simulink model "imu"  (R2014b)
settings: Solver=FixedStepDiscrete  StartTime=0.0  StopTime=inf  FixedStep=sample_time  RelTol=1e-3
settings Model: xpc_rtwmakecfg_data=_xpcethercatlib_  SimulationMode=external  BufferReuse=off  Creator=wmartin  LastModifiedBy=drl
settings SolverCC: EnableConcurrentExecution=on
settings DataIOCC: MaxDataPoints=1000000000  SaveFormat=StructureWithTime  SaveOutput=off  SaveTime=off
settings OptimizationCC: BlockReduction=off  OptimizeBlockIOStorage=off  BufferReuse=off  GlobalBufferReuse=off  ExpressionFolding=off  ExpressionDepthLimit=2147483647  LocalBlockOutputs=off  SimCompilerOptimization=On
settings DebuggingCC: ArtificialAlgebraicLoopMsg=none  UnderspecifiedInitializationDetection=Classic  MergeDetectMultiDrivingBlocksExec=none  StateNameClashWarn=warning
settings HardwareCC: ProdIntDivRoundTo=Zero  ProdEndianess=LittleEndian  ProdLongLongMode=on  ProdHWDeviceType=Generic->32-bit x86 compatible
settings ModelReferenceCC: EnableParallelModelReferenceBuilds=on  ModelReferenceNumInstancesAllowed=Single  ModelReferenceMinAlgLoopOccurrences=on
settings RTWCC: SystemTargetFile=slrt.tlc  TemplateMakefile=slrt_default_tmf  Description=Simulink Real-Time  RTWVerbose=off  ProcessScript=slrt_make_rtw_hook  RTWCompilerOptimization=On
settings CodeAppCC: MaxIdLength=256
settings SimulinkRealTimeCC: GeneratePreprocessorConditionals=Disable all  EnableShiftOperators=on  RL32LogBufSizeModifier=100000000

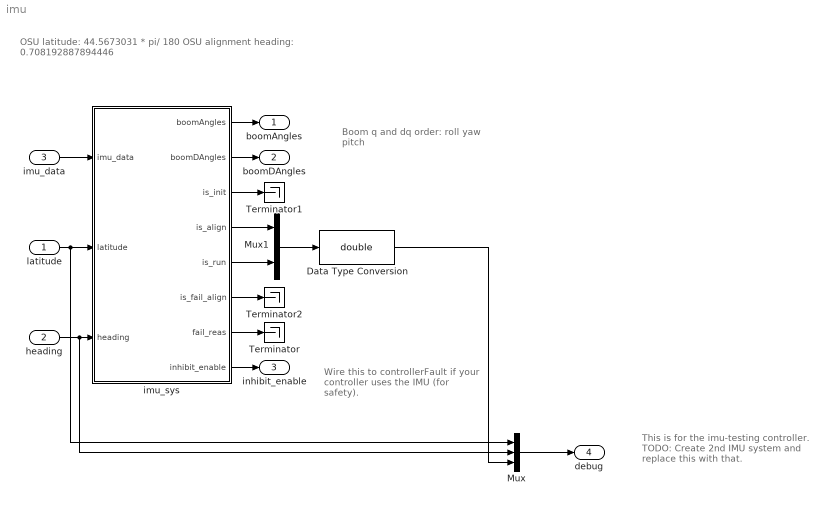
== system imu ==
  note: Wire this to controllerFault
      | if your controller uses the IMU
      | (for safety).
  note: This is for the imu-testing controller.
      | TODO: Create 2nd IMU system and
      | replace this with that.
  note: Boom q and dq order:
      | 	roll
      | 	yaw
      | 	pitch
  note: OSU latitude: 44.5673031 * pi/ 180
      | OSU alignment heading: 0.708192887894446
  latitude : Inport
  heading : Inport  Port=2
  imu_data : Inport  Port=3
  Data Type Conversion : DataTypeConversion  OutDataTypeStr=double
  Mux : Mux  Inputs=3
  Mux1 : Mux  Inputs=2
  Terminator : Terminator
  Terminator1 : Terminator
  Terminator2 : Terminator
  imu_sys : MATLAB Function  TreatAsAtomicUnit=on
  boomAngles : Outport
  boomDAngles : Outport  Port=2
  inhibit_enable : Outport  Port=3
  debug : Outport  Port=4
  wires:
  imu_data/1 -> imu_sys/1(imu_data)
  heading/1 -> Mux/2, imu_sys/3(heading)
  latitude/1 -> imu_sys/2(latitude), Mux/1
  imu_sys/1(boomAngles) -> boomAngles/1
  imu_sys/2(boomDAngles) -> boomDAngles/1
  imu_sys/8(inhibit_enable) -> inhibit_enable/1
  imu_sys/7(fail_reas) -> Terminator/1
  imu_sys/6(is_fail_align) -> Terminator2/1
  imu_sys/3(is_init) -> Terminator1/1
  imu_sys/4(is_align) -> Mux1/1
  imu_sys/5(is_run) -> Mux1/2
  Mux1/1 -> Data Type Conversion/1
  Data Type Conversion/1 -> Mux/3
  Mux/1 -> debug/1

== matlab function imu/imu_sys ==
  data: imu_data input size=9; latitude input size=1; heading input size=1; boomAngles output size=[3 1]; boomDAngles output size=[3 1]; sample_time parameter size=1; is_init output size=1; is_align output size=1; is_run output size=1; is_fail_align output size=1; fail_reas output size=1; inhibit_enable output size=1
function [boomAngles,boomDAngles,is_init,is_align,is_run,is_fail_align,fail_reas,inhibit_enable] ...
    = fcn(imu_data, latitude, heading, sample_time)
%#codegen

% All our saved state is in these objects
persistent imu bc
if isempty(imu)
    imu = IMUSys(sample_time);
    bc  = BoomCoords;
end

% Run the IMU and BoomCoords objects
[local_orient, ang_vel, state, fail_reas] = ...
    imu.update(imu_data(1:3), imu_data(4:6), uint8(imu_data(7)), uint8(imu_data(8)), latitude, heading);

[boomRoll, boomPitch, boomYaw, dBoomRoll, dBoomPitch, dBoomYaw] = ...
    bc.update(local_orient, ang_vel);

% Fully define our outputs to make MATLAB happy
boomAngles  = [boomRoll;  boomYaw;  boomPitch ];
boomDAngles = [dBoomRoll; dBoomYaw; dBoomPitch];

% Create some additional diagnostic outputs
is_init       = state == IMUSysState.INIT;
is_align      = state == IMUSysState.ALIGN;
is_run        = state == IMUSysState.RUN;
is_fail_align = state == IMUSysState.FAIL;

% This output can be fed into the estop safeties, and will prevent the
% robot from enabling when IMU data is not available.
inhibit_enable = state ~= IMUSysState.RUN;
